simulink model "yanshou54"  (R2017a)
settings: Solver=VariableStepAuto  StartTime=0.0  StopTime=10.0  RelTol=1e-3
settings Model: Creator=adi  LastModifiedBy=adi

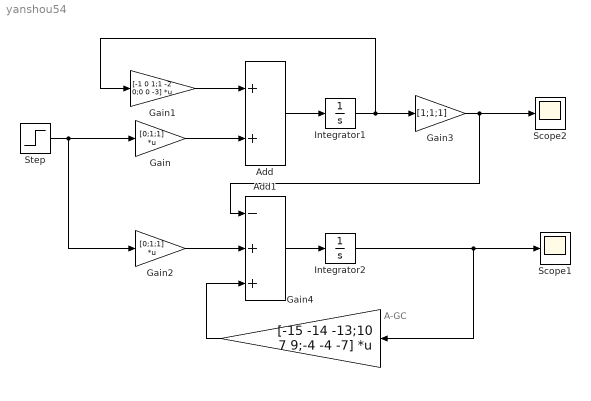
== system yanshou54 ==
  note: A-GC
  Add : Sum
  Add1 : Sum  Inputs=-++
  Gain : Gain  Gain=[0;1;1]  Multiplication=Matrix(K*u)
  Gain1 : Gain  Gain=[-1 0 1;1 -2 0;0 0 -3]  Multiplication=Matrix(K*u)
  Gain2 : Gain  Gain=[0;1;1]  Multiplication=Matrix(K*u)
  Gain3 : Gain  Gain=[1;1;1]
  Gain4 : Gain  Gain=[-15 -14 -13;10 7 9;-4 -4 -7]  Multiplication=Matrix(K*u)
  Integrator1 : Integrator
  Integrator2 : Integrator
  Scope1 : Scope
  Scope2 : Scope
  Step : Step  SampleTime=0
  wires:
  Step/1 -> Gain2/1, Gain/1
  Gain/1 -> Add/2
  Gain1/1 -> Add/1
  Add/1 -> Integrator1/1
  Integrator1/1 -> Gain3/1, Gain1/1
  Gain3/1 -> Add1/1, Scope2/1
  Gain2/1 -> Add1/2
  Add1/1 -> Integrator2/1
  Gain4/1 -> Add1/3
  Integrator2/1 -> Scope1/1, Gain4/1
